simulink model "MPC_try1"  (R2020b)
settings: Solver=ode15s  StartTime=0.0  StopTime=1.5  RelTol=1e-3
values from neighbouring files (symbols this model uses):
  I_mat = [I_xx I_xy I_xz ... (first row only)    [AngularDynamics_VV.m]    (also in angular_tune_test.m; temp.m)
libraries: cstblocks x2, mpclib x1
settings Model: Creator=Jonathan van Zyl  LastModifiedBy=Jonathan van Zyl
settings SolverCC: ZeroCrossControl=EnableAll

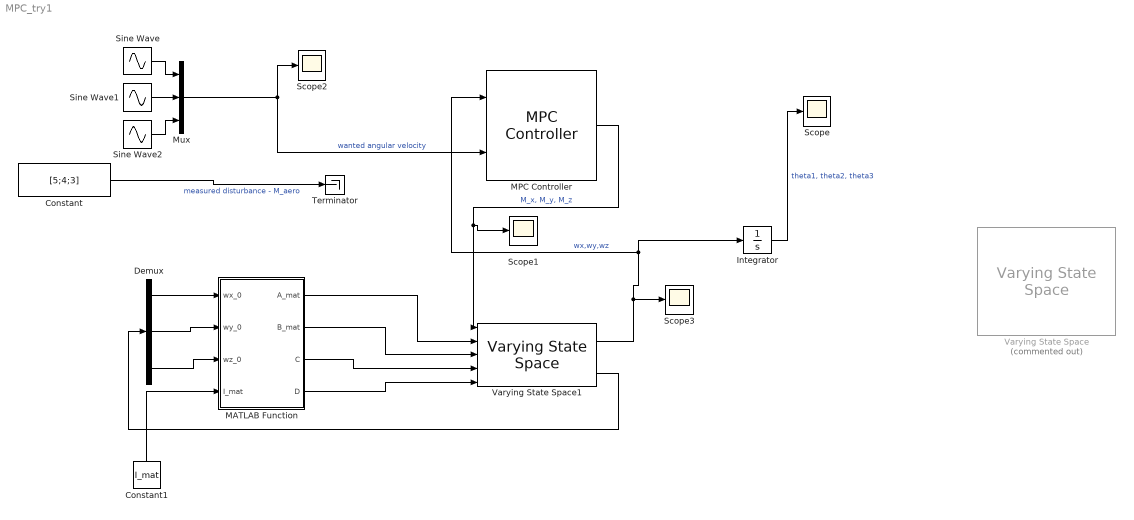
== system MPC_try1 ==
  Constant : Constant  Value=[5;4;3]
  Constant1 : Constant  Value=I_mat
  Demux : Demux  Outputs=3
  Integrator : Integrator
  MATLAB Function : MATLAB Function  TreatAsAtomicUnit=on
  MPC Controller : mpclib/MPC Controller  SCDEnableBlockLinearizationSpecification=on  is_multiple=0  enable_value=0  return_u0=off  updateMPCinCallerWorkspace=on  md_inport=off  mv_inport=off  uref_inport=off  return_cost=off  return_mvseq=off  return_qpstatus=off  return_xseq=off  return_state=off  return_ovseq=off  state_inport=off  umin_inport=off  umax_inport=off  ymin_inport=off  ymax_inport=off  cc_inport=off  ywt_inport=off  uwt_inport=off  duwt_inport=off  rhoeps_inport=off  pm_inport=off  MaximumP=10  HorizonChoice=FixedHorizon  n_ts=0.1  n_p=10  n_mv=3  n_md=1  n_ud=0  n_mo=3  n_uo=0  BlockDataType=double  SampleTimeInherited=off  switch_inport=off
  Mux : Mux  Inputs=3
  Scope{,1..3} (4 alike) : Scope
  Sine Wave : Sin  SampleTime=0
  Sine Wave1 : Sin  Amplitude=0.5  Frequency=0.7  SampleTime=0
  Sine Wave2 : Sin  Amplitude=4  Frequency=0.5  SampleTime=0
  Terminator : Terminator
  Varying State Space : cstblocks/Linear Parameter Varying/Varying State Space  Commented=on  x0=0  xNames=''  OutputX=on  OutputDX=off
  Varying State Space1 : cstblocks/Linear Parameter Varying/Varying State Space  x0=0  xNames=''  OutputX=on  OutputDX=off
  wires:
  MPC Controller/1 -> Varying State Space1/1, Scope1/1  "M_x, M_y, M_z"
  MATLAB Function/1(A_mat) -> Varying State Space1/2
  MATLAB Function/2(B_mat) -> Varying State Space1/3
  MATLAB Function/3(C) -> Varying State Space1/4
  MATLAB Function/4(D) -> Varying State Space1/5
  Varying State Space1/2 -> Demux/1
  Demux/1 -> MATLAB Function/1(wx_0)
  Demux/2 -> MATLAB Function/2(wy_0)
  Demux/3 -> MATLAB Function/3(wz_0)
  Constant1/1 -> MATLAB Function/4(I_mat)
  Varying State Space1/1 -> Integrator/1, MPC Controller/1, Scope3/1  "wx,wy,wz"
  Integrator/1 -> Scope/1  "theta1, theta2, theta3"
  Mux/1 -> MPC Controller/2, Scope2/1  "wanted angular velocity"
  Constant/1 -> Terminator/1  "measured disturbance - M_aero"
  Sine Wave2/1 -> Mux/3
  Sine Wave1/1 -> Mux/2
  Sine Wave/1 -> Mux/1

== matlab function MPC_try1/MATLAB Function ==
  data: wx_0 input; A_mat output; wy_0 input; wz_0 input; I_mat input; B_mat output; C output; D output
function[A_mat, B_mat, C, D] = func(wx_0, wy_0, wz_0, I_mat)
I_xx = I_mat(1,1);
I_xy = I_mat(1,2);
I_xz = I_mat(1,3);

I_yx = I_mat(2,1);
I_yy = I_mat(2,2);
I_yz = I_mat(2,3);

I_zx = I_mat(3,1);
I_zy = I_mat(3,2);
I_zz = I_mat(3,3);
%% Calculate A matrix
%Calculate numerators
a = (I_yy*I_zz - I_yz*I_zy)*(I_zx*wy_0 - I_yx*wz_0) + (I_xx*I_zy - I_xy*I_zz)*(I_xx*wz_0 - I_zx*wy_0 - I_zz*wz_0) + (I_xy*I_yz - I_xz*I_yy)*(I_zx*wx_0 + I_zy*wy_0 + I_zz*wz_0 - I_yx*wy_0);
b = (I_yy*I_zz - I_yz*I_zy)*(I_zx*wx_0 + I_zy*wy_0 + I_zz*wz_0 - I_yy*wz_0) + (I_xz*I_zy - I_xy*I_zz)*(I_xy*wz_0 - I_zz*wx_0) + (I_xy*I_yz - I_xz*I_yy)*(I_zz*wx_0 - I_yx*wx_0 - I_yy*wy_0 - I_yz*wz_0);
c = (I_yy*I_zz - I_yz*I_zy)*(I_zz*wy_0 - I_yx*wx_0 - I_yy*wy_0 - I_yz*wz_0) + (I_xz*I_zy - I_xy*I_zz)*(I_xx*wx_0 + I_xy*wy_0 + I_xz*wz_0 - I_zz*wx_0) + (I_xy*I_yz - I_xz*I_yy)*(I_zz*wx_0 - I_yz*wy_0);
d = (I_yz*I_zx - I_yx*I_zz)*(I_zx*wy_0 - I_yx*wz_0) + (I_xx*I_zz - I_xz*I_zx)*(I_xx*wz_0 - I_zx*wx_0 - I_zy*wy_0 - I_zz*wz_0) + (I_xz*I_yx - I_xx*I_yz)*(I_zx*wx_0 + I_zz*wz_0 - I_yx*wy_0);
e = (I_yz*I_zx - I_yx*I_zz)*(I_zx*wx_0 + I_zy*wy_0 + I_zz*wz_0 - I_yy*wz_0) + (I_xx*I_zz - I_xz*I_zx)*(I_xy*wz_0 - I_zz*wz_0) + (I_xz*I_yx - I_xx*I_yz)*(I_zz*wx_0 - I_yx*wx_0 - I_yy*wy_0 - I_yz*wz_0);
f = (I_yz*I_zx - I_yx*I_zz)*(I_zz*wy_0 - I_yx*wx_0 - I_yy*wy_0 -I_yz*wz_0) + (I_xx*I_zz - I_xz*I_zx)*(I_xx*wx_0 + I_xy*wy_0 + I_xz*wz_0 - I_zz*wx_0) + (I_xz*I_yx - I_xx*I_yz)*(I_zz*wx_0 - I_yz*wy_0);
g = (I_yx*I_zy - I_yy*I_zx)*(I_zx*wy_0 - I_yx*wz_0) + (I_xy*I_zx - I_xx*I_zy)*(I_xx*wz_0 - I_zx*wx_0 - I_zy*wy_0 - I_zz*wz_0) + (I_xx*I_yy - I_xy*I_yx)*(I_zx*wx_0 + I_zy*wy_0 + I_zz*wz_0 - I_yx*wy_0);
h = (I_yx*I_zy - I_yy*I_zx)*(I_zx*wx_0 + I_zy*wy_0 + I_zz*wz_0 - I_yy*wz_0) + (I_xy*I_zx - I_xx*I_zy)*(I_xy*wz_0 - I_zz*wx_0) + (I_xx*I_yy - I_xy*I_yx)*(I_zz*wx_0 - I_yx*wx_0 - I_yy*wy_0 - I_yz*wz_0);
i = (I_yx*I_zy - I_yy*I_zx)*(I_zz*wy_0 - I_yx*wx_0 - I_yy*wy_0 - I_yz*wz_0) + (I_xy*I_zx - I_xx*I_zy)*(I_xx*wx_0 + I_xy*wy_0 + I_xz*wz_0 - I_zz*wx_0) + (I_xx*I_yy - I_xy*I_yx)*(I_zz*wx_0 - I_yz*wy_0);
%Calculate denominator
A_d= I_xx*I_yy*I_zz + I_xy*I_yz*I_zx + I_xz*I_yx*I_zy - I_zx*I_yy*I_xz - I_zy*I_yz*I_xx - I_zz*I_yx*I_xy;
%Form A-matrix
A_mat = [a/A_d b/A_d c/A_d;
    d/A_d e/A_d f/A_d;
    g h i;];

%% Calculate B-matrix
ab = (I_yy*I_zz - I_yz*I_zy)/A_d;
bb = (I_xz*I_zy - I_xy*I_zz)/A_d;
cb = (I_xy*I_yz - I_xz*I_yy)/A_d;
db = (I_yz*I_zx - I_yx*I_zz)/A_d;
eb = (I_xx*I_zz - I_xz*I_zx)/A_d;
fb = (I_xz*I_yx - I_xx*I_yz)/A_d;
gb = (I_yx*I_zy - I_yy*I_zx)/A_d;
hb = (I_xy*I_zx - I_xx*I_zy)/A_d;
ib = (I_xx*I_yy - I_zy*I_yx)/A_d;

B_mat = [ab bb cb;
    db eb fb;
    gb hb ib;];

%% Make C & D matrix

C = eye(3);
D = zeros(3);
end
